simulink model "ConstantFireangle"  (R2021a)
settings: Solver=VariableStepAuto  StartTime=0.0  StopTime=100  RelTol=1e-3
libraries: spsThyristorLib x8, spsACVoltageSourceLib x2, spsDiodeLib x2, spsGroundLib x2, spsDCMachineLib x1, spsIdealSwitchLib x1, spsVoltageMeasurementLib x1, spspowerguiLib x1
settings Model: Creator=User  LastModifiedBy=User

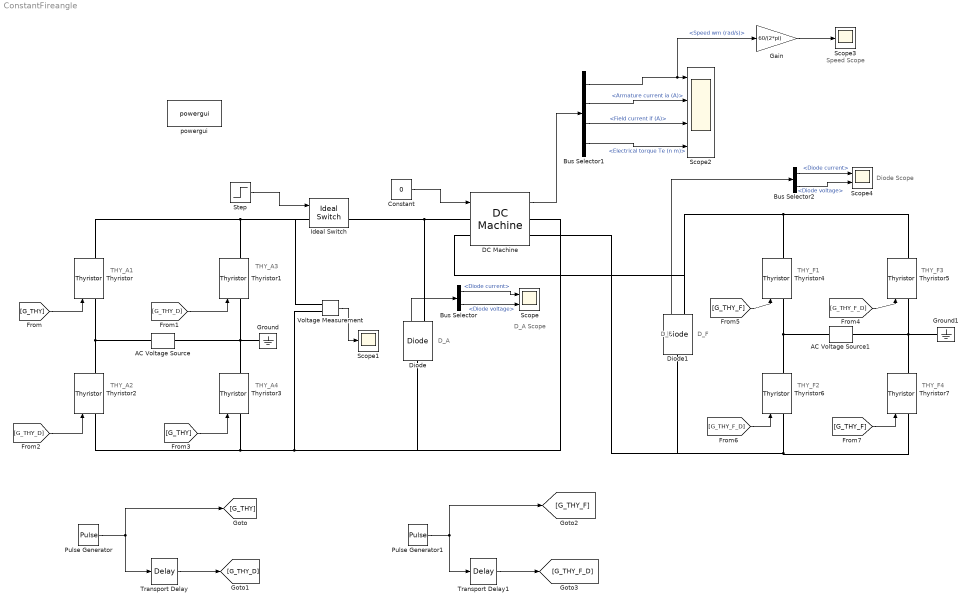
== system ConstantFireangle ==
  note: Diode Scope
  note: Speed Scope
  note: THY_F4
  note: THY_F3
  note: THY_F2
  note: THY_F1
  note: D_F
  note: D_F
  note: D_A Scope
  note: D_A
  note: THY_A4
  note: THY_A2
  note: THY_A3
  note: THY_A1
  AC Voltage Source : spsACVoltageSourceLib/AC Voltage Source  Amplitude=311  Phase=0  Frequency=50  SampleTime=0  Measurements=None  BusType=swing  Pref=10e3  Qref=0  Qmin=-inf  Qmax=+inf
  AC Voltage Source1 : spsACVoltageSourceLib/AC Voltage Source  Amplitude=311  Phase=0  Frequency=50  SampleTime=0  Measurements=None  BusType=swing  Pref=10e3  Qref=0  Qmin=-inf  Qmax=+inf
  Bus Selector : BusSelector  OutputSignals=Diode current,Diode voltage
  Bus Selector1 : BusSelector  OutputSignals=Speed wm (rad/s),Armature current ia (A),Field current if (A),Electrical torque Te (n m)
  Bus Selector2 : BusSelector  OutputSignals=Diode current,Diode voltage
  Constant : Constant  Value=0
  DC Machine : spsDCMachineLib/DC Machine  PresetModel=04: 10HP 240V 1750RPM Field:300V  MechanicalLoad=Torque TL  FieldType=Wound  ShowDetailedParameters=on  MeasurementBus=off  RLa=[1.086 0.01216]  RLf=[180 71.47]  Laf=0.6458  MachineConstant=Torque constant (N.m/A)  Ke=1.8  Kt=1.8  J=0.04251  Bm=0.003406  Tf=1.046  w0=1  Ifinit=8.59463218144815e-18  TsPowergui=0  TsBlock=-1
  Diode : spsDiodeLib/Diode  Ron=0.001  Lon=0  Vf=0.8  IC=0  UseSnubber=0  Rs=500  Cs=250e-9  Measurements=on
  Diode1 : spsDiodeLib/Diode  Ron=0.001  Lon=0  Vf=0.8  IC=0  UseSnubber=0  Rs=500  Cs=250e-9  Measurements=on
  Gain : Gain  Gain=60/(2*pi)
  Ground : spsGroundLib/Ground  LConnTagsString=a
  Ground1 : spsGroundLib/Ground  LConnTagsString=a
  Ideal Switch : spsIdealSwitchLib/Ideal Switch  Ron=0.001  Lon=0  IC=0  Rs=1e5  Cs=inf  Measurements=on
  Pulse Generator : DiscretePulseGenerator  PulseType=Time based  Period=0.02  PulseWidth=5  PhaseDelay=60*0.02/360
  Pulse Generator1 : DiscretePulseGenerator  PulseType=Time based  Period=0.02  PulseWidth=5  PhaseDelay=30*0.02/360
  Scope : Scope  NumInputPorts=2
  Scope1 : Scope
  Scope2 : Scope  NumInputPorts=4
  Scope3 : Scope
  Scope4 : Scope  NumInputPorts=2
  Step : Step  Time=5  SampleTime=0
  Thyristor{,1..7} (8 alike) : spsThyristorLib/Thyristor  Ron=0.001  Lon=0  Vf=0.8  IC=0  Rs=500  Cs=250e-9  Measurements=on
  Transport Delay : TransportDelay  DelayTime=0.01
  Transport Delay1 : TransportDelay  DelayTime=0.01
  Voltage Measurement : spsVoltageMeasurementLib/Voltage Measurement  PhasorSimulation=off  OutputType=Complex  PSBequivalent=0
  powergui : spspowerguiLib/powergui  Priority=1  SimulationMode=Discrete  SampleTime=0.0001  frequency=60  Iterations=50  frequencyindice=50  Pbase=100e6  ErrMax=1e-4  UnitsV=kV  UnitsW=MW  buscounter=0  FunctionMessages=off  echomessages=off  EnableUseOfTLC=off  CurrentSourceSwitches=off  DisableSnubberDevices=off  DisableRonSwitches=off  DisableVfSwitches=off  DisplayEquations=off  AutomaticDiscreteSolvers=off  SolverType=Tustin/Backward Euler (TBE)  Interpol=off  ExternalGateDelay=off  methode=off  Ts=100  x0status=blocks  SPID=on  SwTol=0  HookPort=off  NonlinearTolerance=1e-4  nMaxIteration=100  ContinueOnMaxIteration=off  RestoreLinks=warning  ResistiveCurrentMeasurement=off  Frange=[0:2:500]  Ylog=off  Xlog=on  ShowGrid=off  save=off  variable=ZData  structure=0  ZoomFFT=off  StartTime=0.0  cycles=1  DisplayStyle=1  fundamental=60  FreqAxis=off  MaxFrequency=1000  frequencyindicesteady=1  RmsSteady=1  display=off
  wires:
  [G_THY] -> Thyristor/1
  [G_THY_D] -> Thyristor1/1
  [G_THY_D] -> Thyristor2/1
  [G_THY] -> Thyristor3/1
  Step/1 -> Ideal Switch/1
  Constant/1 -> DC Machine/1
  Diode/1 -> Bus Selector/1
  Bus Selector/1 -> Scope/1  "<Diode current>"
  Bus Selector/2 -> Scope/2  "<Diode voltage>"
  Voltage Measurement/1 -> Scope1/1
  DC Machine/1 -> Bus Selector1/1
  Bus Selector1/1 -> Scope2/1, Gain/1  "<Speed wm (rad/s)>"
  Bus Selector1/2 -> Scope2/2  "<Armature current ia (A)>"
  Gain/1 -> Scope3/1
  Diode1/1 -> Bus Selector2/1
  Bus Selector2/1 -> Scope4/1  "<Diode current>"
  Bus Selector2/2 -> Scope4/2  "<Diode voltage>"
  [G_THY_F_D] -> Thyristor5/1
  [G_THY_F] -> Thyristor4/1
  [G_THY_F_D] -> Thyristor6/1
  [G_THY_F] -> Thyristor7/1
  Transport Delay/1 -> [G_THY_D]
  Pulse Generator/1 -> Transport Delay/1, [G_THY]
  Transport Delay1/1 -> [G_THY_F_D]
  Pulse Generator1/1 -> Transport Delay1/1, [G_THY_F]
  Bus Selector1/3 -> Scope2/3  "<Field current if (A)>"
  Bus Selector1/4 -> Scope2/4  "<Electrical torque Te (n m)>"
  connections:
  Thyristor2/RConn1 -- Thyristor/LConn1 -- AC Voltage Source/RConn1
  Thyristor1/LConn1 -- AC Voltage Source/LConn1 -- Ground/LConn1 -- Thyristor3/RConn1
  Thyristor/RConn1 -- Voltage Measurement/LConn1 -- Ideal Switch/LConn1 -- Thyristor1/RConn1
  Thyristor2/LConn1 -- DC Machine/RConn1 -- Diode/LConn1 -- Voltage Measurement/LConn2 -- Thyristor3/LConn1
  DC Machine/LConn1 -- Diode/RConn1 -- Ideal Switch/RConn1
  Thyristor4/LConn1 -- Thyristor6/RConn1 -- AC Voltage Source1/RConn1
  Thyristor5/LConn1 -- Ground1/LConn1 -- AC Voltage Source1/LConn1 -- Thyristor7/RConn1
  Thyristor4/RConn1 -- DC Machine/LConn2 -- Diode1/RConn1 -- Thyristor5/RConn1
  Thyristor6/LConn1 -- DC Machine/RConn2 -- Diode1/LConn1 -- Thyristor7/LConn1
